simulink model "model324"  (R2024b)
settings: Solver=VariableStepAuto  StartTime=0.0  StopTime=10.0  RelTol=1e-3
undefined symbols (not defined in the file): K1, K2, obj1, obj2, thr, X01, X02, X1d, X1d_dot, X2d, X2d_dot, X3d, X3d_dot
libraries: slctrl_constraint x1
settings Model: Creator=dorec  LastModifiedBy=Filippo
settings OptimizationCC: ReuseModelBlockBuffer=off
settings RTWCC: GPUComputeCapability=3.5

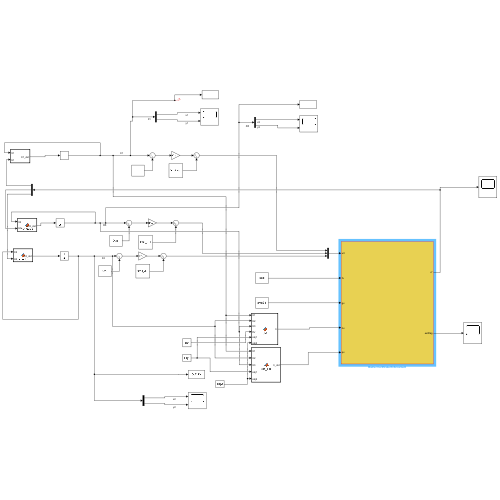
[thumbnail: Simulink's stored preview of the top-level diagram]
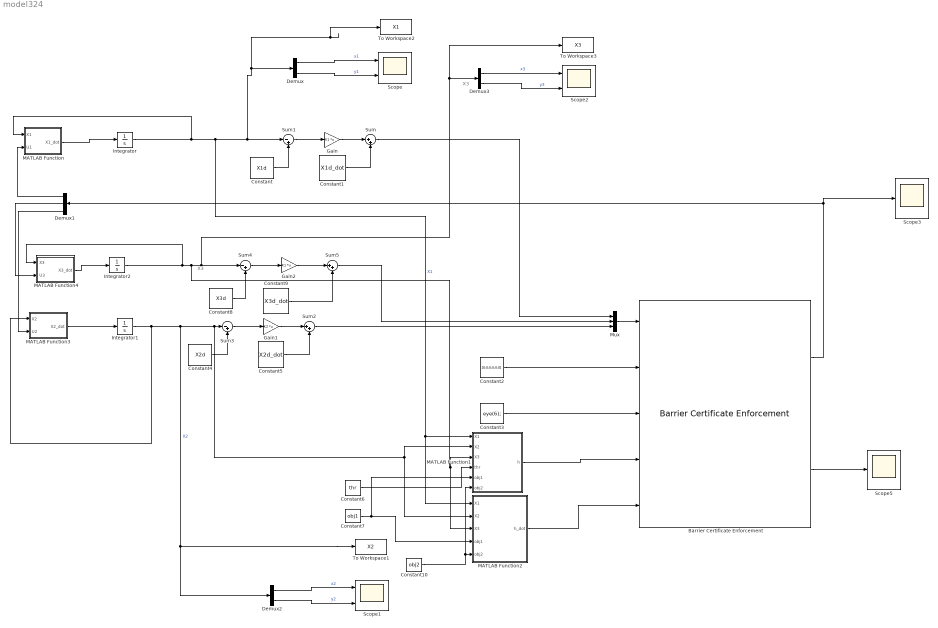
== system model324 ==
  note: X3
  note: X3
  Barrier Certificate Enforcement : slctrl_constraint/Barrier Certificate Enforcement  nx=6  nu=6  nc=9  gamma=10  beta=1  external_umax=off  external_umin=off  Ts=0.1  maxiter=200  tol=1e-6  output_exitflag=on
      settings: LibrarySourceBlock=slctrlblks/Constraint Control/Barrier Certificate Enforcement
  Constant : Constant  Value=X1d
  Constant1 : Constant  Value=X1d_dot
  Constant10 : Constant  Value=obj2
  Constant2 : Constant  Value=[0;0;0;0;0;0]
  Constant3 : Constant  Value=eye(6);
  Constant4 : Constant  Value=X2d
  Constant5 : Constant  Value=X2d_dot
  Constant6 : Constant  Value=thr
  Constant7 : Constant  Value=obj1
  Constant8 : Constant  Value=X3d
  Constant9 : Constant  Value=X3d_dot
  Demux : Demux  Outputs=2
  Demux1 : Demux  Outputs=3
  Demux2 : Demux  Outputs=2
  Demux3 : Demux  Outputs=2
  Gain : Gain  Gain=K1  Multiplication=Matrix(K*u)
  Gain1 : Gain  Gain=K2  Multiplication=Matrix(K*u)
  Gain2 : Gain  Gain=K1  Multiplication=Matrix(K*u)
  Integrator : Integrator  InitialCondition=X01
  Integrator1 : Integrator  InitialCondition=X02
  Integrator2 : Integrator  InitialCondition=X02
  MATLAB Function : MATLAB Function  TreatAsAtomicUnit=on
  MATLAB Function1 : MATLAB Function  TreatAsAtomicUnit=on
  MATLAB Function2 : MATLAB Function  TreatAsAtomicUnit=on
  MATLAB Function3 : MATLAB Function  TreatAsAtomicUnit=on
  MATLAB Function4 : MATLAB Function  TreatAsAtomicUnit=on
  Mux : Mux  Inputs=3
  Scope : Scope  NumInputPorts=2
  Scope1 : Scope  NumInputPorts=2
  Scope2 : Scope  NumInputPorts=2
  Scope3 : Scope
  Scope5 : Scope
  Sum : Sum  Inputs=|++
  Sum1 : Sum  Inputs=|-+
  Sum2 : Sum  Inputs=|++
  Sum3 : Sum  Inputs=|-+
  Sum4 : Sum  Inputs=|-+
  Sum5 : Sum  Inputs=|++
  To Workspace1 : ToWorkspace  VariableName=X2  SaveFormat=Timeseries  SampleTime=-1
  To Workspace2 : ToWorkspace  VariableName=X1  SaveFormat=Timeseries  SampleTime=-1
  To Workspace3 : ToWorkspace  VariableName=X3  SaveFormat=Timeseries  SampleTime=-1
  wires:
  Integrator/1 -> MATLAB Function2/1(X1), MATLAB Function1/1(X1), Sum1/1, To Workspace2/1, Demux/1, MATLAB Function/1(X1)  "X1"
  Sum1/1 -> Gain/1
  Constant/1 -> Sum1/2
  Gain/1 -> Sum/1
  Constant1/1 -> Sum/2
  Sum/1 -> Mux/1
  MATLAB Function/1(X1_dot) -> Integrator/1
  Demux/1 -> Scope/1  "x1"
  Demux/2 -> Scope/2  "y1"
  MATLAB Function1/1(h) -> Barrier Certificate Enforcement/4
  MATLAB Function2/1(h_dot) -> Barrier Certificate Enforcement/5
  Constant3/1 -> Barrier Certificate Enforcement/3
  Constant2/1 -> Barrier Certificate Enforcement/2
  Barrier Certificate Enforcement/1 -> Scope3/1, Demux1/1
  Constant5/1 -> Sum2/2
  Constant4/1 -> Sum3/2
  Gain1/1 -> Sum2/1
  Sum3/1 -> Gain1/1
  Integrator1/1 -> MATLAB Function3/1(X2), To Workspace1/1, Demux2/1, MATLAB Function2/2(X2), MATLAB Function1/2(X2), Sum3/1  "X2"
  MATLAB Function3/1(X2_dot) -> Integrator1/1
  Sum2/1 -> Mux/3
  Mux/1 -> Barrier Certificate Enforcement/1
  Demux1/1 -> MATLAB Function/2(U1)
  Demux1/3 -> MATLAB Function3/2(U2)
  Demux2/1 -> Scope1/1  "x2"
  Demux2/2 -> Scope1/2  "y2"
  Barrier Certificate Enforcement/2 -> Scope5/1
  Constant6/1 -> MATLAB Function1/4(thr)
  Constant7/1 -> MATLAB Function2/4(obj1), MATLAB Function1/5(obj1)
  MATLAB Function4/1(X3_dot) -> Integrator2/1
  Integrator2/1 -> MATLAB Function4/1(X3), MATLAB Function2/3(X3), MATLAB Function1/3(X3), To Workspace3/1, Demux3/1, Sum4/1
  Sum4/1 -> Gain2/1
  Constant8/1 -> Sum4/2
  Gain2/1 -> Sum5/1
  Constant9/1 -> Sum5/2
  Demux1/2 -> MATLAB Function4/2(U3)
  Sum5/1 -> Mux/2
  Demux3/2 -> Scope2/2  "y3"
  Demux3/1 -> Scope2/1  "x3"
  Constant10/1 -> MATLAB Function2/5(obj2), MATLAB Function1/6(obj2)

== matlab function model324/MATLAB Function1 ==
  data: X1 input; X2 input; X3 input; thr input; h output; obj1 input; obj2 input
function h = cbf(X1, X2, X3, thr, obj1, obj2)

    % --- Robot–Robot ---
    h12 = norm(X1 - X2) - thr;
    h13 = norm(X1 - X3) - thr;
    h23 = norm(X2 - X3) - thr;

    % --- Robot–Ostacolo 1 ---
    h1o1 = norm(X1 - obj1) - thr;
    h2o1 = norm(X2 - obj1) - thr;
    h3o1 = norm(X3 - obj1) - thr;

    % --- Robot–Ostacolo 2 ---
    h1o2 = norm(X1 - obj2) - thr;
    h2o2 = norm(X2 - obj2) - thr;
    h3o2 = norm(X3 - obj2) - thr;

    % Output come vettore (tutti i vincoli)
    h = [h12; h13; h23; h1o1; h2o1; h3o1; h1o2; h2o2; h3o2];
end

== matlab function model324/MATLAB Function ==
  data: X1 input; U1 input size=[2 1]; X1_dot output
function X1_dot = dynamics(X1,U1)

x1_dot = U1(1);
y1_dot = U1(2);

X1_dot = [x1_dot; y1_dot];

== matlab function model324/MATLAB Function2 ==
  data: X1 input; X2 input; X3 input; obj1 input; h_dot output; obj2 input
function h_dot = cbf_dot(X1, X2, X3, obj1, obj2)

    % Normalizza funzioni helper
    n12 = (X1 - X2)/norm(X1 - X2);
    n13 = (X1 - X3)/norm(X1 - X3);
    n23 = (X2 - X3)/norm(X2 - X3);

    n1o1 = (X1 - obj1)/norm(X1 - obj1);
    n2o1 = (X2 - obj1)/norm(X2 - obj1);
    n3o1 = (X3 - obj1)/norm(X3 - obj1);

    n1o2 = (X1 - obj2)/norm(X1 - obj2);
    n2o2 = (X2 - obj2)/norm(X2 - obj2);
    n3o2 = (X3 - obj2)/norm(X3 - obj2);

    % Ogni riga: gradiente di un vincolo h rispetto a [X1; X2; X3]
    h_dot = [
        n12(1) n12(2) -n12(1) -n12(2)   0       0;    % R1-R2
        n13(1) n13(2)    0       0    -n13(1) -n13(2); % R1-R3
        0      0        n23(1) n23(2) -n23(1) -n23(2); % R2-R3

        n1o1(1) n1o1(2)  0 0 0 0; % R1-obj1
        0 0 n2o1(1) n2o1(2) 0 0; % R2-obj1
        0 0 0 0 n3o1(1) n3o1(2); % R3-obj1

        n1o2(1) n1o2(2)  0 0 0 0; % R1-obj2
        0 0 n2o2(1) n2o2(2) 0 0; % R2-obj2
        0 0 0 0 n3o2(1) n3o2(2); % R3-obj2
    ];
end

== matlab function model324/MATLAB Function3 ==
  data: X2 input; U2 input size=[2 1]; X2_dot output
function X2_dot = dynamics(X2,U2)

x2_dot = U2(1);
y2_dot = U2(2);

X2_dot = [x2_dot; y2_dot];

== matlab function model324/MATLAB Function4 ==
  data: X3 input; U3 input size=[2 1]; X3_dot output
function X3_dot = dynamics(X3,U3)

x3_dot = U3(1);
y3_dot = U3(2);

X3_dot = [x3_dot; y3_dot];
